simulink model "CurrentSystem2019a"  (R2019a)
settings: Solver=ode23tb  StartTime=0  StopTime=24*365*60*60  RelTol=0.1  EnableMultiTasking=on
PreLoadFcn:
  | power_13NodeTestFeeder_init;
undefined symbols (not defined in the file): ABSOLARCap, ABWindCap, BCSOLARCap, BCWindCap, C_601, C_602, C_603, C_604, C_605, C_606, C_607, ft2km, L_601, L_602, L_603, L_604, L_605, L_606, L_607, MBSOLARCap, MBWindCap, NBSOLARCap, NBWindCap, NLSOLARCap, NLWindCap, NSSOLARCap, NSWindCap, NTSOLARCap, NTWindCap, NUSOLARCap, NUWindCap, ONSOLARCap, ONWindCap, PEISOLARCap, PEIWindCap, QCSOLARCap, QCWindCap, R_601, R_602, R_603, R_604, R_605, R_606, R_607, SKSOLARCap, SKWindCap, T_Disconnect, T_Reconnect, Yearsec, YTSOLARCap, YTWindCap
libraries: powerlib_meascontrol x70, powerlib x67, sps_avr x1, spsDieselMotorModel x1
(part 2 of 3)

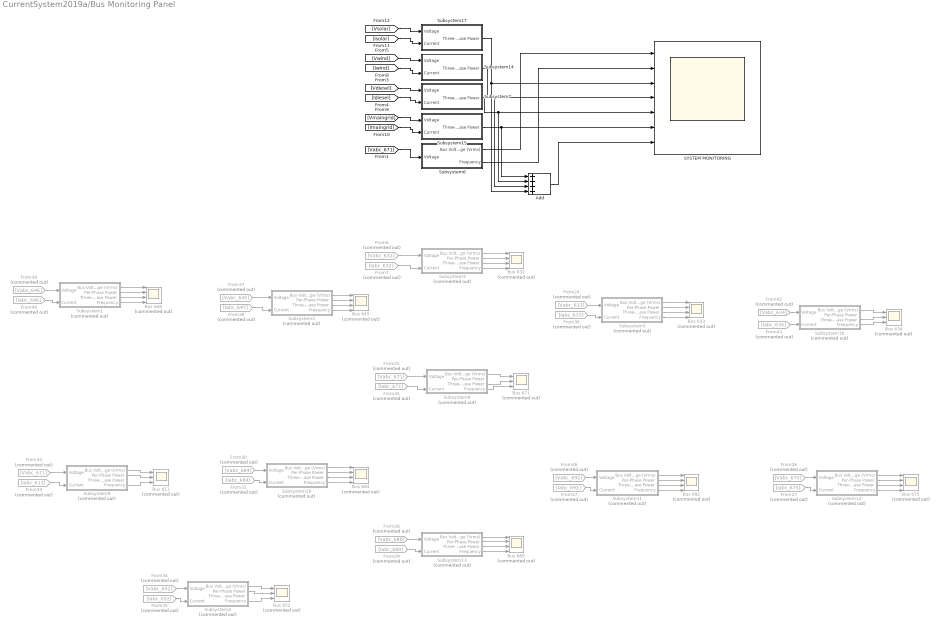
== system CurrentSystem2019a/Bus Monitoring Panel ==
  Add : Sum  Inputs=++++
  Bus {611,634,652,671} (4 alike) : Scope  Commented=on  NumInputPorts=3
  Bus {632..633,645..646,675,680,684,692} (8 alike) : Scope  Commented=on  NumInputPorts=4
  From24 : From  Commented=on  GotoTag=Vabc_633  TagVisibility=global
  From25 : From  Commented=on  GotoTag=Vabc_671  TagVisibility=global
  From26 : From  Commented=on  GotoTag=Vabc_675  TagVisibility=global
  From27 : From  Commented=on  GotoTag=Iabc_675  TagVisibility=global
  From28 : From  Commented=on  GotoTag=Vabc_680  TagVisibility=global
  From29 : From  Commented=on  GotoTag=Iabc_680  TagVisibility=global
  From30 : From  Commented=on  GotoTag=Vabc_684  TagVisibility=global
  From31 : From  Commented=on  GotoTag=Iabc_684  TagVisibility=global
  From32 : From  Commented=on  GotoTag=Vabc_611  TagVisibility=global
  From33 : From  Commented=on  GotoTag=Iabc_611  TagVisibility=global
  From34 : From  Commented=on  GotoTag=Vabc_652  TagVisibility=global
  From35 : From  Commented=on  GotoTag=Iabc_652  TagVisibility=global
  From36 : From  Commented=on  GotoTag=Iabc_633  TagVisibility=global
  From37 : From  Commented=on  GotoTag=Vabc_645  TagVisibility=global
  From38 : From  Commented=on  GotoTag=Iabc_645  TagVisibility=global
  From39 : From  Commented=on  GotoTag=Vabc_646  TagVisibility=global
  From40 : From  Commented=on  GotoTag=Iabc_646  TagVisibility=global
  From41 : From  Commented=on  GotoTag=Iabc_671  TagVisibility=global
  From42 : From  Commented=on  GotoTag=Vabc_634  TagVisibility=global
  From43 : From  Commented=on  GotoTag=Iabc_634  TagVisibility=global
  From46 : From  Commented=on  GotoTag=Vabc_692  TagVisibility=global
  From47 : From  Commented=on  GotoTag=Iabc_692  TagVisibility=global
  From6 : From  Commented=on  GotoTag=Vabc_632  TagVisibility=global
  From7 : From  Commented=on  GotoTag=Iabc_632  TagVisibility=global
  SYSTEM MONITORING : Scope  NumInputPorts=7
  Subsystem1 : Subsystem  Commented=on
  Subsystem10 : Subsystem  Commented=on
  Subsystem11 : Subsystem  Commented=on
  Subsystem12 : Subsystem  Commented=on
  Subsystem13 : Subsystem  Commented=on
  Subsystem14 : Subsystem
  Subsystem15 : Subsystem
  Subsystem16 : Subsystem  Commented=on
  Subsystem17 : Subsystem
  Subsystem2 : Subsystem  Commented=on
  Subsystem3 : Subsystem  Commented=on
  Subsystem4 : Subsystem  Commented=on
  Subsystem5 : Subsystem  Commented=on
  Subsystem6 : Subsystem
  Subsystem7 : Subsystem
  Subsystem8 : Subsystem  Commented=on
  Subsystem9 : Subsystem  Commented=on
  wires:
  From37/1 -> Subsystem2/1(Voltage)
  From43/1 -> Subsystem16/2(Current)
  From42/1 -> Subsystem16/1(Voltage)
  Subsystem5/3(Three-Phase Power) -> Bus 633/3
  Subsystem5/1(Bus Voltage (Vrms)) -> Bus 633/1
  Subsystem5/2(Per-Phase Power) -> Bus 633/2
  Subsystem5/4(Frequency) -> Bus 633/4
  From24/1 -> Subsystem5/1(Voltage)
  From36/1 -> Subsystem5/2(Current)
  Subsystem3/4(Frequency) -> Bus 632/4
  Subsystem3/1(Bus Voltage (Vrms)) -> Bus 632/1
  Subsystem3/2(Per-Phase Power) -> Bus 632/2
  Subsystem3/3(Three-Phase Power) -> Bus 632/3
  From6/1 -> Subsystem3/1(Voltage)
  From7/1 -> Subsystem3/2(Current)
  Subsystem2/4(Frequency) -> Bus 645/4
  Subsystem2/1(Bus Voltage (Vrms)) -> Bus 645/1
  Subsystem2/2(Per-Phase Power) -> Bus 645/2
  Subsystem2/3(Three-Phase Power) -> Bus 645/3
  From38/1 -> Subsystem2/2(Current)
  Subsystem1/4(Frequency) -> Bus 646/4
  Subsystem1/1(Bus Voltage (Vrms)) -> Bus 646/1
  Subsystem1/2(Per-Phase Power) -> Bus 646/2
  Subsystem1/3(Three-Phase Power) -> Bus 646/3
  From39/1 -> Subsystem1/1(Voltage)
  From40/1 -> Subsystem1/2(Current)
  From25/1 -> Subsystem8/1(Voltage)
  From41/1 -> Subsystem8/2(Current)
  From32/1 -> Subsystem9/1(Voltage)
  From33/1 -> Subsystem9/2(Current)
  Subsystem10/4(Frequency) -> Bus 684/4
  Subsystem10/1(Bus Voltage (Vrms)) -> Bus 684/1
  Subsystem10/2(Per-Phase Power) -> Bus 684/2
  Subsystem10/3(Three-Phase Power) -> Bus 684/3
  From30/1 -> Subsystem10/1(Voltage)
  From31/1 -> Subsystem10/2(Current)
  Subsystem11/4(Frequency) -> Bus 692/4
  Subsystem11/1(Bus Voltage (Vrms)) -> Bus 692/1
  Subsystem11/2(Per-Phase Power) -> Bus 692/2
  Subsystem11/3(Three-Phase Power) -> Bus 692/3
  From46/1 -> Subsystem11/1(Voltage)
  From47/1 -> Subsystem11/2(Current)
  Subsystem12/4(Frequency) -> Bus 675/4
  Subsystem12/1(Bus Voltage (Vrms)) -> Bus 675/1
  Subsystem12/2(Per-Phase Power) -> Bus 675/2
  Subsystem12/3(Three-Phase Power) -> Bus 675/3
  From26/1 -> Subsystem12/1(Voltage)
  From27/1 -> Subsystem12/2(Current)
  Subsystem13/4(Frequency) -> Bus 680/4
  Subsystem13/1(Bus Voltage (Vrms)) -> Bus 680/1
  Subsystem13/2(Per-Phase Power) -> Bus 680/2
  Subsystem13/3(Three-Phase Power) -> Bus 680/3
  From28/1 -> Subsystem13/1(Voltage)
  From29/1 -> Subsystem13/2(Current)
  From34/1 -> Subsystem4/1(Voltage)
  From35/1 -> Subsystem4/2(Current)
  Subsystem9/1(Bus Voltage (Vrms)) -> Bus 611/1
  Subsystem9/2(Per-Phase Power) -> Bus 611/2
  Subsystem9/4(Frequency) -> Bus 611/3
  Subsystem4/1(Bus Voltage (Vrms)) -> Bus 652/1
  Subsystem4/2(Per-Phase Power) -> Bus 652/2
  Subsystem4/4(Frequency) -> Bus 652/3
  [Vabc_671] -> Subsystem6/1(Voltage)
  Subsystem16/1(Bus Voltage (Vrms)) -> Bus 634/1
  Subsystem16/3(Three-Phase Power) -> Bus 634/2
  Subsystem16/4(Frequency) -> Bus 634/3
  [Idiesel] -> Subsystem7/2(Current)
  [Vdiesel] -> Subsystem7/1(Voltage)
  [Iwind] -> Subsystem14/2(Current)
  [Vwind] -> Subsystem14/1(Voltage)
  Subsystem8/1(Bus Voltage (Vrms)) -> Bus 671/1
  Subsystem8/3(Three-Phase Power) -> Bus 671/2
  Subsystem8/4(Frequency) -> Bus 671/3
  [Vmaingrid] -> Subsystem15/1(Voltage)
  [Imaingrid] -> Subsystem15/2(Current)
  [Isolar] -> Subsystem17/2(Current)
  [Vsolar] -> Subsystem17/1(Voltage)
  Subsystem6/1(Bus Voltage (Vrms)) -> SYSTEM MONITORING/1
  Subsystem6/2(Frequency) -> SYSTEM MONITORING/2
  Subsystem17/1(Three-Phase Power) -> Add/4, SYSTEM MONITORING/3
  Subsystem14/1(Three-Phase Power) -> Add/3, SYSTEM MONITORING/4
  Subsystem7/1(Three-Phase Power) -> Add/2, SYSTEM MONITORING/5
  Subsystem15/1(Three-Phase Power) -> Add/1, SYSTEM MONITORING/6
  Add/1 -> SYSTEM MONITORING/7

== system CurrentSystem2019a/Diesel Generator1 ==
  wref (pu) : Inport
  Vref (pu) : Inport  Port=2
  AC1A Excitation System : sps_avr/AC1A Excitation System  Tr=20e-3  KaTa=[400 .02]  VAminmax=[-14.5 14.5]  VRminmax=[-5.43 6.03]  KfTf=[0.03 1]  TbTc=[0 0]  KeTe=[1 0.8]  Ve12=[4.18 3.14]  SeVe12=[0.1 0.03]  Kd=0.38  Kc=0.2  v0=[1.0249 1.0264]  TsBlock=0
      link override Model/Saturation Vx=Ve*Se[Ve]/Saturation: BeginIndexSearchUsingPreviousIndexResult=on
      settings: SourceProductName=Simscape Electrical  SourceProductBaseCode=PS
  Diesel Engine Governor : spsDieselMotorModel/Diesel Engine Governor  K=29  Tr=[0.01 0.02 0.2]  Ta=[0.25 0.009 0.0384]  Tlim=[0 1.1]  Td=0.024  Pm0=0.050009
      settings: SourceProductName=Simscape Electrical  SourceProductBaseCode=PS
  Generator Measures : Subsystem
  Ground : Ground
  Selected Measurements : Subsystem
  Synchronous Machine : powerlib/Machines/Synchronous Machine pu Standard  PresetModel=No  MechanicalLoad=Mechanical power Pm  ShowDetailedParameters=on  RotorType=Salient-pole  Units=per unit standard parameters  MeasurementBus=off  NominalParameters=[ Pn Vn Fn]  Reactances1=[ 1.81, 0.3, 0.23, 1.76, 0.65, 0.25, 0.15 ]  Reactances2=[1.305 0.296 0.252 0.474 0.243 0.18]  dAxisTimeConstants=Open-circuit  qAxisTimeConstants=Short-circuit  TimeConstants1="[ 4.4849  0.0681  0.1  ]"  TimeConstants2=[ 8.0, 0.03, 1.0, 0.07 ]  TimeConstants3="[  4.49  0.0681  0.0513  ]"  TimeConstants4=[ 8.0, 0.03, 0.3371, 0.0295 ]  TimeConstants5=[ 1.01, 0.053, 0.1 ]  TimeConstants6=[ 1.3201, 0.023, 1.0, 0.07 ]  TimeConstants7=[0.012 0.003 0.003]  TimeConstants8=[ 1.3201, 0.0231, 0.3371, 0.0295 ]  StatorResistance=0.003  Mechanical=[3.7 0 1 ]  PolePairs=20  InitialConditions=[0 -90.7831 0.0390782 0.045527 0.0753264 -35.3217 -89.6639 115.267 1.02644]  SetSaturation=off  Saturation=[0.6404,0.7127,0.8441,0.9214,0.9956,1.082,1.19,1.316,1.457;0.7,0.7698,0.8872,0.9466,0.9969,1.046,1.1,1.151,1.201]  LoadFlowParameters=[1 0 0 0 0]  TsPowergui=0  TsBlock=-1  IterativeModel=Trapezoidal non iterative  IterativeDiscreteModel=Trapezoidal non iterative  BusType=PQ  Pref=Pn*P0  Qref=0  Qmin=-inf  Qmax=inf  PLF=0  QLF=0
      settings: SourceProductName=Simscape Electrical
  A : PMIOPort  Side=Right
  B : PMIOPort  Port=2  Side=Right
  C : PMIOPort  Port=3  Side=Right
  m : Outport
  wires:
  wref (pu)/1 -> Diesel Engine Governor/1
  Diesel Engine Governor/1 -> Synchronous Machine/1
  AC1A Excitation System/1 -> Synchronous Machine/2
  Vref (pu)/1 -> AC1A Excitation System/1
  Synchronous Machine/1 -> Generator Measures/1(m), Selected Measurements/1(m)
  Ground/1 -> AC1A Excitation System/4
  Generator Measures/3(wm) -> Diesel Engine Governor/2
  Generator Measures/2(Vt) -> AC1A Excitation System/2
  Generator Measures/1(Ifd) -> AC1A Excitation System/3
  Selected Measurements/1(sm) -> m/1
  connections:
  A/RConn1 -- Synchronous Machine/RConn1
  B/RConn1 -- Synchronous Machine/RConn2
  C/RConn1 -- Synchronous Machine/RConn3

== system CurrentSystem2019a/MB SOLAR PROFILE ==
  Add : Sum  Inputs=++++++++++++
  Apr : Step  Time=3*Yearsec  After=136-132  SampleTime=0
  Aug : Step  Time=7*Yearsec  After=122-127  SampleTime=0
  Dec : Step  Time=11*Yearsec  After=64-66  SampleTime=0
  Egen : Gain  Gain=MBSOLARCap
  Feb : Step  Time=1*Yearsec  After=106  SampleTime=0
  Jan : Step  Time=1*Yearsec  Before=79  After=0  SampleTime=0
  Jul : Step  Time=6*Yearsec  After=127-124  SampleTime=0
  Jun : Step  Time=5*Yearsec  After=124-127  SampleTime=0
  Mar : Step  Time=2*Yearsec  After=132-106  SampleTime=0
  May : Step  Time=4*Yearsec  After=127-136  SampleTime=0
  Nov : Step  Time=10*Yearsec  After=66-85  SampleTime=0
  Oct : Step  Time=9*Yearsec  After=85-103  SampleTime=0
  Pgen : Gain  Gain=(1/(30*24))*MBSOLARCap
  Sept : Step  Time=8*Yearsec  After=103-122  SampleTime=0
  Energy : Outport
  Power : Outport  Port=2
  wires:
  Dec/1 -> Add/12
  Sept/1 -> Add/9
  Jun/1 -> Add/6
  Nov/1 -> Add/11
  Aug/1 -> Add/8
  Mar/1 -> Add/3
  May/1 -> Add/5
  Apr/1 -> Add/4
  Jan/1 -> Add/1
  Oct/1 -> Add/10
  Jul/1 -> Add/7
  Feb/1 -> Add/2
  Pgen/1 -> Power/1
  Egen/1 -> Energy/1
  Add/1 -> Egen/1, Pgen/1

== system CurrentSystem2019a/MB WIND PROFILE ==
  Add : Sum  Inputs=++++++++++++
  Apr : Step  Time=3*Yearsec  After=165.6-139.2  SampleTime=0
  Aug : Step  Time=7*Yearsec  After=64.8-72  SampleTime=0
  Dec : Step  Time=11*Yearsec  After=127.2-144  SampleTime=0
  Egen : Gain  Gain=MBWindCap
  Feb : Step  Time=1*Yearsec  After=110.4  SampleTime=0
  Jan : Step  Time=1*Yearsec  Before=127.2  After=0  SampleTime=0
  Jul : Step  Time=6*Yearsec  After=72-104.4  SampleTime=0
  Jun : Step  Time=5*Yearsec  After=104.4-127.2  SampleTime=0
  Mar : Step  Time=2*Yearsec  After=139.2-110.4  SampleTime=0
  May : Step  Time=4*Yearsec  After=127.2-165.5  SampleTime=0
  Nov : Step  Time=10*Yearsec  After=144-180  SampleTime=0
  Oct : Step  Time=9*Yearsec  After=180-110.4  SampleTime=0
  Pgen : Gain  Gain=(1/(30*24))*MBWindCap
  Sept : Step  Time=8*Yearsec  After=110.4-64.8  SampleTime=0
  Energy : Outport
  Power : Outport  Port=2
  wires:
  Dec/1 -> Add/12
  Sept/1 -> Add/9
  Jun/1 -> Add/6
  Nov/1 -> Add/11
  Aug/1 -> Add/8
  Mar/1 -> Add/3
  May/1 -> Add/5
  Apr/1 -> Add/4
  Jan/1 -> Add/1
  Oct/1 -> Add/10
  Jul/1 -> Add/7
  Feb/1 -> Add/2
  Pgen/1 -> Power/1
  Egen/1 -> Energy/1
  Add/1 -> Egen/1, Pgen/1

== system CurrentSystem2019a/NB SOLAR PROFILE ==
  Add : Sum  Inputs=++++++++++++
  Apr : Step  Time=3*Yearsec  After=105-113  SampleTime=0
  Aug : Step  Time=7*Yearsec  After=113-112  SampleTime=0
  Dec : Step  Time=11*Yearsec  After=60-60  SampleTime=0
  Egen : Gain  Gain=NBSOLARCap
  Feb : Step  Time=1*Yearsec  After=96  SampleTime=0
  Jan : Step  Time=1*Yearsec  Before=78  After=0  SampleTime=0
  Jul : Step  Time=6*Yearsec  After=112-111  SampleTime=0
  Jun : Step  Time=5*Yearsec  After=111-109  SampleTime=0
  Mar : Step  Time=2*Yearsec  After=113-96  SampleTime=0
  May : Step  Time=4*Yearsec  After=109-105  SampleTime=0
  Nov : Step  Time=10*Yearsec  After=60-83  SampleTime=0
  Oct : Step  Time=9*Yearsec  After=83-103  SampleTime=0
  Pgen : Gain  Gain=(1/(30*24))*NBSOLARCap
  Sept : Step  Time=8*Yearsec  After=103-113  SampleTime=0
  Energy : Outport
  Power : Outport  Port=2
  wires:
  Dec/1 -> Add/12
  Sept/1 -> Add/9
  Jun/1 -> Add/6
  Nov/1 -> Add/11
  Aug/1 -> Add/8
  Mar/1 -> Add/3
  May/1 -> Add/5
  Apr/1 -> Add/4
  Jan/1 -> Add/1
  Oct/1 -> Add/10
  Jul/1 -> Add/7
  Feb/1 -> Add/2
  Pgen/1 -> Power/1
  Egen/1 -> Energy/1
  Add/1 -> Egen/1, Pgen/1

== system CurrentSystem2019a/NB WIND PROFILE ==
  Add : Sum  Inputs=++++++++++++
  Apr : Step  Time=3*Yearsec  After=64.8-91.2  SampleTime=0
  Aug : Step  Time=7*Yearsec  After=0-9.6  SampleTime=0
  Dec : Step  Time=11*Yearsec  After=24-57.6  SampleTime=0
  Egen : Gain  Gain=NBWindCap
  Feb : Step  Time=1*Yearsec  After=50.4  SampleTime=0
  Jan : Step  Time=1*Yearsec  Before=50.4  After=0  SampleTime=0
  Jul : Step  Time=6*Yearsec  After=9.6-24  SampleTime=0
  Jun : Step  Time=5*Yearsec  After=24-60  SampleTime=0
  Mar : Step  Time=2*Yearsec  After=91.2-50.4  SampleTime=0
  May : Step  Time=4*Yearsec  After=60-64.8  SampleTime=0
  Nov : Step  Time=10*Yearsec  After=57.6-24  SampleTime=0
  Oct : Step  Time=9*Yearsec  After=24-9.6  SampleTime=0
  Pgen : Gain  Gain=(1/(30*24))*NBWindCap
  Sept : Step  Time=8*Yearsec  After=9.6-0  SampleTime=0
  Energy : Outport
  Power : Outport  Port=2
  wires:
  Dec/1 -> Add/12
  Sept/1 -> Add/9
  Jun/1 -> Add/6
  Nov/1 -> Add/11
  Aug/1 -> Add/8
  Mar/1 -> Add/3
  May/1 -> Add/5
  Apr/1 -> Add/4
  Jan/1 -> Add/1
  Oct/1 -> Add/10
  Jul/1 -> Add/7
  Feb/1 -> Add/2
  Pgen/1 -> Power/1
  Egen/1 -> Energy/1
  Add/1 -> Egen/1, Pgen/1

== system CurrentSystem2019a/NL SOLAR PROFILE ==
  Add : Sum  Inputs=++++++++++++
  Apr : Step  Time=3*Yearsec  After=96-95  SampleTime=0
  Aug : Step  Time=7*Yearsec  After=99-103  SampleTime=0
  Dec : Step  Time=11*Yearsec  After=38-44  SampleTime=0
  Egen : Gain  Gain=NLSOLARCap
  Feb : Step  Time=1*Yearsec  After=75  SampleTime=0
  Jan : Step  Time=1*Yearsec  Before=51  After=0  SampleTime=0
  Jul : Step  Time=6*Yearsec  After=103-100  SampleTime=0
  Jun : Step  Time=5*Yearsec  After=100-98  SampleTime=0
  Mar : Step  Time=2*Yearsec  After=95-75  SampleTime=0
  May : Step  Time=4*Yearsec  After=98-96  SampleTime=0
  Nov : Step  Time=10*Yearsec  After=44-63  SampleTime=0
  Oct : Step  Time=9*Yearsec  After=63-85  SampleTime=0
  Pgen : Gain  Gain=(1/(30*24))*NLSOLARCap
  Sept : Step  Time=8*Yearsec  After=85-99  SampleTime=0
  Energy : Outport
  Power : Outport  Port=2
  wires:
  Dec/1 -> Add/12
  Sept/1 -> Add/9
  Jun/1 -> Add/6
  Nov/1 -> Add/11
  Aug/1 -> Add/8
  Mar/1 -> Add/3
  May/1 -> Add/5
  Apr/1 -> Add/4
  Jan/1 -> Add/1
  Oct/1 -> Add/10
  Jul/1 -> Add/7
  Feb/1 -> Add/2
  Pgen/1 -> Power/1
  Egen/1 -> Energy/1
  Add/1 -> Egen/1, Pgen/1

== system CurrentSystem2019a/NL WIND PROFILE ==
  Add : Sum  Inputs=++++++++++++
  Apr : Step  Time=3*Yearsec  After=408-420  SampleTime=0
  Aug : Step  Time=7*Yearsec  After=168-216  SampleTime=0
  Dec : Step  Time=11*Yearsec  After=516-336  SampleTime=0
  Egen : Gain  Gain=NLWindCap
  Feb : Step  Time=1*Yearsec  After=552  SampleTime=0
  Jan : Step  Time=1*Yearsec  Before=420  After=0  SampleTime=0
  Jul : Step  Time=6*Yearsec  After=216-264  SampleTime=0
  Jun : Step  Time=5*Yearsec  After=264-264  SampleTime=0
  Mar : Step  Time=2*Yearsec  After=420-552  SampleTime=0
  May : Step  Time=4*Yearsec  After=264-408  SampleTime=0
  Nov : Step  Time=10*Yearsec  After=336-264  SampleTime=0
  Oct : Step  Time=9*Yearsec  After=264-228  SampleTime=0
  Pgen : Gain  Gain=(1/(30*24))*NLWindCap
  Sept : Step  Time=8*Yearsec  After=228-168  SampleTime=0
  Energy : Outport
  Power : Outport  Port=2
  wires:
  Dec/1 -> Add/12
  Sept/1 -> Add/9
  Jun/1 -> Add/6
  Nov/1 -> Add/11
  Aug/1 -> Add/8
  Mar/1 -> Add/3
  May/1 -> Add/5
  Apr/1 -> Add/4
  Jan/1 -> Add/1
  Oct/1 -> Add/10
  Jul/1 -> Add/7
  Feb/1 -> Add/2
  Pgen/1 -> Power/1
  Egen/1 -> Energy/1
  Add/1 -> Egen/1, Pgen/1

== system CurrentSystem2019a/NS SOLAR PROFILE ==
  Add : Sum  Inputs=++++++++++++
  Apr : Step  Time=3*Yearsec  After=98-105  SampleTime=0
  Aug : Step  Time=7*Yearsec  After=111-111  SampleTime=0
  Dec : Step  Time=11*Yearsec  After=52-56  SampleTime=0
  Egen : Gain  Gain=NSSOLARCap
  Feb : Step  Time=1*Yearsec  After=89  SampleTime=0
  Jan : Step  Time=1*Yearsec  Before=66  After=0  SampleTime=0
  Jul : Step  Time=6*Yearsec  After=111-112  SampleTime=0
  Jun : Step  Time=5*Yearsec  After=112-106  SampleTime=0
  Mar : Step  Time=2*Yearsec  After=105-89  SampleTime=0
  May : Step  Time=4*Yearsec  After=106-98  SampleTime=0
  Nov : Step  Time=10*Yearsec  After=56-82  SampleTime=0
  Oct : Step  Time=9*Yearsec  After=82-102  SampleTime=0
  Pgen : Gain  Gain=(1/(30*24))*NSSOLARCap
  Sept : Step  Time=8*Yearsec  After=102-111  SampleTime=0
  Energy : Outport
  Power : Outport  Port=2
  wires:
  Dec/1 -> Add/12
  Sept/1 -> Add/9
  Jun/1 -> Add/6
  Nov/1 -> Add/11
  Aug/1 -> Add/8
  Mar/1 -> Add/3
  May/1 -> Add/5
  Apr/1 -> Add/4
  Jan/1 -> Add/1
  Oct/1 -> Add/10
  Jul/1 -> Add/7
  Feb/1 -> Add/2
  Pgen/1 -> Power/1
  Egen/1 -> Energy/1
  Add/1 -> Egen/1, Pgen/1

== system CurrentSystem2019a/NS WIND PROFILE ==
  Add : Sum  Inputs=++++++++++++
  Apr : Step  Time=3*Yearsec  After=66-96  SampleTime=0
  Aug : Step  Time=7*Yearsec  After=0-0  SampleTime=0
  Dec : Step  Time=11*Yearsec  After=69.6-72  SampleTime=0
  Egen : Gain  Gain=NSWindCap
  Feb : Step  Time=1*Yearsec  After=72  SampleTime=0
  Jan : Step  Time=1*Yearsec  Before=91.2  After=0  SampleTime=0
  Jul : Step  Time=6*Yearsec  After=0-12  SampleTime=0
  Jun : Step  Time=5*Yearsec  After=12-20.4  SampleTime=0
  Mar : Step  Time=2*Yearsec  After=96-72  SampleTime=0
  May : Step  Time=4*Yearsec  After=20.4-66  SampleTime=0
  Nov : Step  Time=10*Yearsec  After=72-45.6  SampleTime=0
  Oct : Step  Time=9*Yearsec  After=45.6-13.2  SampleTime=0
  Pgen : Gain  Gain=(1/(30*24))*NSWindCap
  Sept : Step  Time=8*Yearsec  After=13.2-0  SampleTime=0
  Energy : Outport
  Power : Outport  Port=2
  wires:
  Dec/1 -> Add/12
  Sept/1 -> Add/9
  Jun/1 -> Add/6
  Nov/1 -> Add/11
  Aug/1 -> Add/8
  Mar/1 -> Add/3
  May/1 -> Add/5
  Apr/1 -> Add/4
  Jan/1 -> Add/1
  Oct/1 -> Add/10
  Jul/1 -> Add/7
  Feb/1 -> Add/2
  Pgen/1 -> Power/1
  Egen/1 -> Energy/1
  Add/1 -> Egen/1, Pgen/1

== system CurrentSystem2019a/NT SOLAR PROFILE ==
  Add : Sum  Inputs=++++++++++++
  Apr : Step  Time=3*Yearsec  After=98-105  SampleTime=0
  Aug : Step  Time=7*Yearsec  After=111-111  SampleTime=0
  Dec : Step  Time=11*Yearsec  After=52-56  SampleTime=0
  Egen : Gain  Gain=NTSOLARCap
  Feb : Step  Time=1*Yearsec  After=89  SampleTime=0
  Jan : Step  Time=1*Yearsec  Before=66  After=0  SampleTime=0
  Jul : Step  Time=6*Yearsec  After=111-112  SampleTime=0
  Jun : Step  Time=5*Yearsec  After=112-106  SampleTime=0
  Mar : Step  Time=2*Yearsec  After=105-89  SampleTime=0
  May : Step  Time=4*Yearsec  After=106-98  SampleTime=0
  Nov : Step  Time=10*Yearsec  After=56-82  SampleTime=0
  Oct : Step  Time=9*Yearsec  After=82-102  SampleTime=0
  Pgen : Gain  Gain=(1/(30*24))*NTSOLARCap
  Scope : Scope
  Sept : Step  Time=8*Yearsec  After=102-111  SampleTime=0
  Energy : Outport
  Power : Outport  Port=2
  wires:
  Dec/1 -> Add/12
  Sept/1 -> Add/9
  Jun/1 -> Add/6
  Nov/1 -> Add/11
  Aug/1 -> Add/8
  Mar/1 -> Add/3
  May/1 -> Add/5
  Apr/1 -> Add/4
  Jan/1 -> Add/1
  Oct/1 -> Add/10
  Jul/1 -> Add/7
  Feb/1 -> Add/2
  Pgen/1 -> Power/1
  Egen/1 -> Energy/1
  Add/1 -> Scope/1, Egen/1, Pgen/1

== system CurrentSystem2019a/NT WIND PROFILE ==
  Add : Sum  Inputs=++++++++++++
  Apr : Step  Time=3*Yearsec  After=67.2-52.8  SampleTime=0
  Aug : Step  Time=7*Yearsec  After=52.8-63.6  SampleTime=0
  Dec : Step  Time=11*Yearsec  After=24-60  SampleTime=0
  Egen : Gain  Gain=NTWindCap
  Feb : Step  Time=1*Yearsec  After=24  SampleTime=0
  Jan : Step  Time=1*Yearsec  Before=36  After=0  SampleTime=0
  Jul : Step  Time=6*Yearsec  After=63.6-78  SampleTime=0
  Jun : Step  Time=5*Yearsec  After=78-96  SampleTime=0
  Mar : Step  Time=2*Yearsec  After=52.8-24  SampleTime=0
  May : Step  Time=4*Yearsec  After=96-67.2  SampleTime=0
  Nov : Step  Time=10*Yearsec  After=60-60  SampleTime=0
  Oct : Step  Time=9*Yearsec  After=60-84  SampleTime=0
  Pgen : Gain  Gain=(1/(30*24))*NTWindCap
  Sept : Step  Time=8*Yearsec  After=84-52.8  SampleTime=0
  Energy : Outport
  Power : Outport  Port=2
  wires:
  Dec/1 -> Add/12
  Sept/1 -> Add/9
  Jun/1 -> Add/6
  Nov/1 -> Add/11
  Aug/1 -> Add/8
  Mar/1 -> Add/3
  May/1 -> Add/5
  Apr/1 -> Add/4
  Jan/1 -> Add/1
  Oct/1 -> Add/10
  Jul/1 -> Add/7
  Feb/1 -> Add/2
  Pgen/1 -> Power/1
  Egen/1 -> Energy/1
  Add/1 -> Egen/1, Pgen/1

== system CurrentSystem2019a/NU SOLAR PROFILE ==
  Add : Sum  Inputs=++++++++++++
  Apr : Step  Time=3*Yearsec  After=175-153  SampleTime=0
  Aug : Step  Time=7*Yearsec  After=92-111  SampleTime=0
  Dec : Step  Time=11*Yearsec  After=15-34  SampleTime=0
  Egen : Gain  Gain=NUSOLARCap
  Feb : Step  Time=1*Yearsec  After=89  SampleTime=0
  Jan : Step  Time=1*Yearsec  Before=31  After=0  SampleTime=0
  Jul : Step  Time=6*Yearsec  After=111-126  SampleTime=0
  Jun : Step  Time=5*Yearsec  After=126-153  SampleTime=0
  Mar : Step  Time=2*Yearsec  After=153-89  SampleTime=0
  May : Step  Time=4*Yearsec  After=153-175  SampleTime=0
  Nov : Step  Time=10*Yearsec  After=34-51  SampleTime=0
  Oct : Step  Time=9*Yearsec  After=51-64  SampleTime=0
  Pgen : Gain  Gain=(1/(30*24))*NUSOLARCap
  Sept : Step  Time=8*Yearsec  After=64-92  SampleTime=0
  Energy : Outport
  Power : Outport  Port=2
  wires:
  Dec/1 -> Add/12
  Sept/1 -> Add/9
  Jun/1 -> Add/6
  Nov/1 -> Add/11
  Aug/1 -> Add/8
  Mar/1 -> Add/3
  May/1 -> Add/5
  Apr/1 -> Add/4
  Jan/1 -> Add/1
  Oct/1 -> Add/10
  Jul/1 -> Add/7
  Feb/1 -> Add/2
  Pgen/1 -> Power/1
  Egen/1 -> Energy/1
  Add/1 -> Egen/1, Pgen/1

== system CurrentSystem2019a/NU WIND PROFILE ==
  Add : Sum  Inputs=++++++++++++
  Apr : Step  Time=3*Yearsec  After=204-168  SampleTime=0
  Aug : Step  Time=7*Yearsec  After=52.8-60  SampleTime=0
  Dec : Step  Time=11*Yearsec  After=105.6-122.4  SampleTime=0
  Egen : Gain  Gain=NUWindCap
  Feb : Step  Time=1*Yearsec  After=100.8  SampleTime=0
  Jan : Step  Time=1*Yearsec  Before=96  After=0  SampleTime=0
  Jul : Step  Time=6*Yearsec  After=60-67.2  SampleTime=0
  Jun : Step  Time=5*Yearsec  After=67.2-108  SampleTime=0
  Mar : Step  Time=2*Yearsec  After=168-100.8  SampleTime=0
  May : Step  Time=4*Yearsec  After=108-204  SampleTime=0
  Nov : Step  Time=10*Yearsec  After=122.4-104.4  SampleTime=0
  Oct : Step  Time=9*Yearsec  After=104.4-100.8  SampleTime=0
  Pgen : Gain  Gain=(1/(30*24))*NUWindCap
  Sept : Step  Time=8*Yearsec  After=100.8-52.8  SampleTime=0
  Energy : Outport
  Power : Outport  Port=2
  wires:
  Dec/1 -> Add/12
  Sept/1 -> Add/9
  Jun/1 -> Add/6
  Nov/1 -> Add/11
  Aug/1 -> Add/8
  Mar/1 -> Add/3
  May/1 -> Add/5
  Apr/1 -> Add/4
  Jan/1 -> Add/1
  Oct/1 -> Add/10
  Jul/1 -> Add/7
  Feb/1 -> Add/2
  Pgen/1 -> Power/1
  Egen/1 -> Energy/1
  Add/1 -> Egen/1, Pgen/1

== system CurrentSystem2019a/ON SOLAR PROFILE ==
  Add : Sum  Inputs=++++++++++++
  Apr : Step  Time=3*Yearsec  After=115-109  SampleTime=0
  Aug : Step  Time=7*Yearsec  After=118-125  SampleTime=0
  Dec : Step  Time=11*Yearsec  After=52-56  SampleTime=0
  Egen : Gain  Gain=ONSOLARCap
  Feb : Step  Time=1*Yearsec  After=92  SampleTime=0
  Jan : Step  Time=1*Yearsec  Before=66  After=0  SampleTime=0
  Jul : Step  Time=6*Yearsec  After=125-124  SampleTime=0
  Jun : Step  Time=5*Yearsec  After=124-119  SampleTime=0
  Mar : Step  Time=2*Yearsec  After=109-92  SampleTime=0
  May : Step  Time=4*Yearsec  After=119-115  SampleTime=0
  Nov : Step  Time=10*Yearsec  After=56-86  SampleTime=0
  Oct : Step  Time=9*Yearsec  After=86-104  SampleTime=0
  Pgen : Gain  Gain=(1/(30*24))*ONSOLARCap
  Sept : Step  Time=8*Yearsec  After=104-118  SampleTime=0
  Energy : Outport
  Power : Outport  Port=2
  wires:
  Dec/1 -> Add/12
  Sept/1 -> Add/9
  Jun/1 -> Add/6
  Nov/1 -> Add/11
  Aug/1 -> Add/8
  Mar/1 -> Add/3
  May/1 -> Add/5
  Apr/1 -> Add/4
  Jan/1 -> Add/1
  Oct/1 -> Add/10
  Jul/1 -> Add/7
  Feb/1 -> Add/2
  Pgen/1 -> Power/1
  Egen/1 -> Energy/1
  Add/1 -> Egen/1, Pgen/1

== system CurrentSystem2019a/ON WIND PROFILE ==
  Add : Sum  Inputs=++++++++++++
  Apr : Step  Time=3*Yearsec  After=110.4-127.2  SampleTime=0
  Aug : Step  Time=7*Yearsec  After=63.6-67.2  SampleTime=0
  Dec : Step  Time=11*Yearsec  After=110.4-105.6  SampleTime=0
  Egen : Gain  Gain=ONWindCap
  Feb : Step  Time=1*Yearsec  After=160.8  SampleTime=0
  Jan : Step  Time=1*Yearsec  Before=144  After=0  SampleTime=0
  Jul : Step  Time=6*Yearsec  After=67.2-91.2  SampleTime=0
  Jun : Step  Time=5*Yearsec  After=91.2-88.8  SampleTime=0
  Mar : Step  Time=2*Yearsec  After=127.2-160.8  SampleTime=0
  May : Step  Time=4*Yearsec  After=88.8-110.4  SampleTime=0
  Nov : Step  Time=10*Yearsec  After=105.6-96  SampleTime=0
  Oct : Step  Time=9*Yearsec  After=96-60  SampleTime=0
  Pgen : Gain  Gain=(1/(30*24))*ONWindCap
  Sept : Step  Time=8*Yearsec  After=60-63.6  SampleTime=0
  Energy : Outport
  Power : Outport  Port=2
  wires:
  Dec/1 -> Add/12
  Sept/1 -> Add/9
  Jun/1 -> Add/6
  Nov/1 -> Add/11
  Aug/1 -> Add/8
  Mar/1 -> Add/3
  May/1 -> Add/5
  Apr/1 -> Add/4
  Jan/1 -> Add/1
  Oct/1 -> Add/10
  Jul/1 -> Add/7
  Feb/1 -> Add/2
  Pgen/1 -> Power/1
  Egen/1 -> Energy/1
  Add/1 -> Egen/1, Pgen/1

== system CurrentSystem2019a/PEI SOLAR PROFILE ==
  Add : Sum  Inputs=++++++++++++
  Apr : Step  Time=3*Yearsec  After=102-110  SampleTime=0
  Aug : Step  Time=7*Yearsec  After=112-114  SampleTime=0
  Dec : Step  Time=11*Yearsec  After=50-54  SampleTime=0
  Egen : Gain  Gain=PEISOLARCap
  Feb : Step  Time=1*Yearsec  After=94  SampleTime=0
  Jan : Step  Time=1*Yearsec  Before=69  After=0  SampleTime=0
  Jul : Step  Time=6*Yearsec  After=114-114  SampleTime=0
  Jun : Step  Time=5*Yearsec  After=114-109  SampleTime=0
  Mar : Step  Time=2*Yearsec  After=110-94  SampleTime=0
  May : Step  Time=4*Yearsec  After=109-102  SampleTime=0
  Nov : Step  Time=10*Yearsec  After=54-77  SampleTime=0
  Oct : Step  Time=9*Yearsec  After=77-100  SampleTime=0
  Pgen : Gain  Gain=(1/(30*24))*PEISOLARCap
  Sept : Step  Time=8*Yearsec  After=100-112  SampleTime=0
  Energy : Outport
  Power : Outport  Port=2
  wires:
  Dec/1 -> Add/12
  Sept/1 -> Add/9
  Jun/1 -> Add/6
  Nov/1 -> Add/11
  Aug/1 -> Add/8
  Mar/1 -> Add/3
  May/1 -> Add/5
  Apr/1 -> Add/4
  Jan/1 -> Add/1
  Oct/1 -> Add/10
  Jul/1 -> Add/7
  Feb/1 -> Add/2
  Pgen/1 -> Power/1
  Egen/1 -> Energy/1
  Add/1 -> Egen/1, Pgen/1

== system CurrentSystem2019a/PEI WIND PROFILE ==
  Add : Sum  Inputs=++++++++++++
  Apr : Step  Time=3*Yearsec  After=120-163.2  SampleTime=0
  Aug : Step  Time=7*Yearsec  After=64.8-64.8  SampleTime=0
  Dec : Step  Time=11*Yearsec  After=120-163.2  SampleTime=0
  Egen : Gain  Gain=PEIWindCap
  Feb : Step  Time=1*Yearsec  After=160.8  SampleTime=0
  Jan : Step  Time=1*Yearsec  Before=144  After=0  SampleTime=0
  Jul : Step  Time=6*Yearsec  After=64.8-100.8  SampleTime=0
  Jun : Step  Time=5*Yearsec  After=100.8-100.8  SampleTime=0
  Mar : Step  Time=2*Yearsec  After=163.2-160.8  SampleTime=0
  May : Step  Time=4*Yearsec  After=100.8-120  SampleTime=0
  Nov : Step  Time=10*Yearsec  After=163.2-98.4  SampleTime=0
  Oct : Step  Time=9*Yearsec  After=98.4-69.6  SampleTime=0
  Pgen : Gain  Gain=(1/(30*24))*PEIWindCap
  Sept : Step  Time=8*Yearsec  After=69.6-64.8  SampleTime=0
  Energy : Outport
  Power : Outport  Port=2
  wires:
  Dec/1 -> Add/12
  Sept/1 -> Add/9
  Jun/1 -> Add/6
  Nov/1 -> Add/11
  Aug/1 -> Add/8
  Mar/1 -> Add/3
  May/1 -> Add/5
  Apr/1 -> Add/4
  Jan/1 -> Add/1
  Oct/1 -> Add/10
  Jul/1 -> Add/7
  Feb/1 -> Add/2
  Pgen/1 -> Power/1
  Egen/1 -> Energy/1
  Add/1 -> Egen/1, Pgen/1

== system CurrentSystem2019a/QC SOLAR PROFILE ==
  Add : Sum  Inputs=++++++++++++
  Apr : Step  Time=3*Yearsec  After=118-124  SampleTime=0
  Aug : Step  Time=7*Yearsec  After=114-117  SampleTime=0
  Dec : Step  Time=11*Yearsec  After=60-59  SampleTime=0
  Egen : Gain  Gain=QCSOLARCap
  Feb : Step  Time=1*Yearsec  After=106  SampleTime=0
  Jan : Step  Time=1*Yearsec  Before=76  After=0  SampleTime=0
  Jul : Step  Time=6*Yearsec  After=117-115  SampleTime=0
  Jun : Step  Time=5*Yearsec  After=115-117  SampleTime=0
  Mar : Step  Time=2*Yearsec  After=124-106  SampleTime=0
  May : Step  Time=4*Yearsec  After=117-118  SampleTime=0
  Nov : Step  Time=10*Yearsec  After=59-80  SampleTime=0
  Oct : Step  Time=9*Yearsec  After=80-98  SampleTime=0
  Pgen : Gain  Gain=(1/(30*24))*QCSOLARCap
  Sept : Step  Time=8*Yearsec  After=98-114  SampleTime=0
  Energy : Outport
  Power : Outport  Port=2
  wires:
  Dec/1 -> Add/12
  Sept/1 -> Add/9
  Jun/1 -> Add/6
  Nov/1 -> Add/11
  Aug/1 -> Add/8
  Mar/1 -> Add/3
  May/1 -> Add/5
  Apr/1 -> Add/4
  Jan/1 -> Add/1
  Oct/1 -> Add/10
  Jul/1 -> Add/7
  Feb/1 -> Add/2
  Pgen/1 -> Power/1
  Egen/1 -> Energy/1
  Add/1 -> Egen/1, Pgen/1

== system CurrentSystem2019a/QC WIND PROFILE ==
  Add : Sum  Inputs=++++++++++++
  Apr : Step  Time=3*Yearsec  After=96-91.2  SampleTime=0
  Aug : Step  Time=7*Yearsec  After=9.6-14.4  SampleTime=0
  Dec : Step  Time=11*Yearsec  After=66-69.6  SampleTime=0
  Egen : Gain  Gain=QCWindCap
  Feb : Step  Time=1*Yearsec  After=103.2  SampleTime=0
  Jan : Step  Time=1*Yearsec  Before=98.4  After=0  SampleTime=0
  Jul : Step  Time=6*Yearsec  After=14.4-50.4  SampleTime=0
  Jun : Step  Time=5*Yearsec  After=50.4-60  SampleTime=0
  Mar : Step  Time=2*Yearsec  After=91.2-103.2  SampleTime=0
  May : Step  Time=4*Yearsec  After=60-96  SampleTime=0
  Nov : Step  Time=10*Yearsec  After=69.6-57.6  SampleTime=0
  Oct : Step  Time=9*Yearsec  After=57.6-11.52  SampleTime=0
  Pgen : Gain  Gain=(1/(30*24))*QCWindCap
  Sept : Step  Time=8*Yearsec  After=11.52-9.6  SampleTime=0
  Energy : Outport
  Power : Outport  Port=2
  wires:
  Dec/1 -> Add/12
  Sept/1 -> Add/9
  Jun/1 -> Add/6
  Nov/1 -> Add/11
  Aug/1 -> Add/8
  Mar/1 -> Add/3
  May/1 -> Add/5
  Apr/1 -> Add/4
  Jan/1 -> Add/1
  Oct/1 -> Add/10
  Jul/1 -> Add/7
  Feb/1 -> Add/2
  Pgen/1 -> Power/1
  Egen/1 -> Energy/1
  Add/1 -> Egen/1, Pgen/1

== system CurrentSystem2019a/SK SOLAR PROFILE ==
  Add : Sum  Inputs=++++++++++++
  Apr : Step  Time=3*Yearsec  After=135-129  SampleTime=0
  Aug : Step  Time=7*Yearsec  After=129-131  SampleTime=0
  Dec : Step  Time=11*Yearsec  After=67-75  SampleTime=0
  Egen : Gain  Gain=SKSOLARCap
  Feb : Step  Time=1*Yearsec  After=111  SampleTime=0
  Jan : Step  Time=1*Yearsec  Before=81  After=0  SampleTime=0
  Jul : Step  Time=6*Yearsec  After=131-128  SampleTime=0
  Jun : Step  Time=5*Yearsec  After=128-128  SampleTime=0
  Mar : Step  Time=2*Yearsec  After=129-111  SampleTime=0
  May : Step  Time=4*Yearsec  After=128-135  SampleTime=0
  Nov : Step  Time=10*Yearsec  After=75-102  SampleTime=0
  Oct : Step  Time=9*Yearsec  After=102-114  SampleTime=0
  Pgen : Gain  Gain=(1/(30*24))*SKSOLARCap
  Sept : Step  Time=8*Yearsec  After=114-129  SampleTime=0
  Energy : Outport
  Power : Outport  Port=2
  wires:
  Dec/1 -> Add/12
  Sept/1 -> Add/9
  Jun/1 -> Add/6
  Nov/1 -> Add/11
  Aug/1 -> Add/8
  Mar/1 -> Add/3
  May/1 -> Add/5
  Apr/1 -> Add/4
  Jan/1 -> Add/1
  Oct/1 -> Add/10
  Jul/1 -> Add/7
  Feb/1 -> Add/2
  Pgen/1 -> Power/1
  Egen/1 -> Energy/1
  Add/1 -> Egen/1, Pgen/1

== system CurrentSystem2019a/SK WIND PROFILE ==
  Add : Sum  Inputs=++++++++++++
  Apr : Step  Time=3*Yearsec  After=204-192  SampleTime=0
  Aug : Step  Time=7*Yearsec  After=88.8-100.8  SampleTime=0
  Dec : Step  Time=11*Yearsec  After=108-127.2  SampleTime=0
  Egen : Gain  Gain=SKWindCap
  Feb : Step  Time=1*Yearsec  After=96  SampleTime=0
  Jan : Step  Time=1*Yearsec  Before=144  After=0  SampleTime=0
  Jul : Step  Time=6*Yearsec  After=100.8-127.2  SampleTime=0
  Jun : Step  Time=5*Yearsec  After=127.2-163.2  SampleTime=0
  Mar : Step  Time=2*Yearsec  After=192-96  SampleTime=0
  May : Step  Time=4*Yearsec  After=163.2-204  SampleTime=0
  Nov : Step  Time=10*Yearsec  After=127.2-160.8  SampleTime=0
  Oct : Step  Time=9*Yearsec  After=160.8-104.4  SampleTime=0
  Pgen : Gain  Gain=(1/(30*24))*SKWindCap
  Sept : Step  Time=8*Yearsec  After=104.4-88.8  SampleTime=0
  Energy : Outport
  Power : Outport  Port=2
  wires:
  Dec/1 -> Add/12
  Sept/1 -> Add/9
  Jun/1 -> Add/6
  Nov/1 -> Add/11
  Aug/1 -> Add/8
  Mar/1 -> Add/3
  May/1 -> Add/5
  Apr/1 -> Add/4
  Jan/1 -> Add/1
  Oct/1 -> Add/10
  Jul/1 -> Add/7
  Feb/1 -> Add/2
  Pgen/1 -> Power/1
  Egen/1 -> Energy/1
  Add/1 -> Egen/1, Pgen/1

== system CurrentSystem2019a/Solar Array ==
  P : Inport
  Bus Selector : BusSelector  OutputSignals=Active power P (W)
  Constant11 : Constant  Value=0
  Mux1 : Mux  Inputs=2
  Simple Solar Inverter : powerlib/Elements/Three-Phase Dynamic Load  NominalVoltage=[Vn Fn]  ActiveReactivePowers=[-250000 -3.38813e-13]  PositiveSequence=[0.999844 -0.0038635]  ExternalControl=on  NpNq=[1.3 2]  TimeConstants="[0  0  0  0]"  MinimumVoltage=0.7  Tfilter=1e-2  LoadFlowParameters=[4,0,0,0,0]
      settings: SourceProductName=Simscape Electrical  SourceProductBaseCode=PS
  Unary Minus : UnaryMinus
  Unary Minus1 : UnaryMinus
  A : PMIOPort  Side=Right
  B : PMIOPort  Port=2  Side=Right
  C : PMIOPort  Port=3  Side=Right
  m : Outport
  wires:
  P/1 -> Unary Minus/1
  Unary Minus/1 -> Mux1/1
  Mux1/1 -> Simple Solar Inverter/1
  Constant11/1 -> Mux1/2
  Simple Solar Inverter/1 -> Bus Selector/1
  Bus Selector/1 -> Unary Minus1/1  "<Active power P (W)>"
  Unary Minus1/1 -> m/1
  connections:
  Simple Solar Inverter/LConn2 -- B/RConn1
  Simple Solar Inverter/LConn3 -- C/RConn1
  Simple Solar Inverter/LConn1 -- A/RConn1

== system CurrentSystem2019a/Wind Turbine ==
  P : Inport
  Bus Selector : BusSelector  OutputSignals=Active power P (W)
  Constant11 : Constant  Value=0
  Mux1 : Mux  Inputs=2
  Simple Solar Inverter : powerlib/Elements/Three-Phase Dynamic Load  NominalVoltage=[Vn Fn]  ActiveReactivePowers=[-250000 -3.38813e-13]  PositiveSequence=[0.999844 -0.0038635]  ExternalControl=on  NpNq=[1.3 2]  TimeConstants="[0  0  0  0]"  MinimumVoltage=0.7  Tfilter=1e-2  LoadFlowParameters=[4,0,0,0,0]
      settings: SourceProductName=Simscape Electrical  SourceProductBaseCode=PS
  Unary Minus : UnaryMinus
  Unary Minus1 : UnaryMinus
  A : PMIOPort  Side=Right
  B : PMIOPort  Port=2  Side=Right
  C : PMIOPort  Port=3  Side=Right
  m : Outport
  wires:
  P/1 -> Unary Minus/1
  Unary Minus/1 -> Mux1/1
  Mux1/1 -> Simple Solar Inverter/1
  Constant11/1 -> Mux1/2
  Simple Solar Inverter/1 -> Bus Selector/1
  Bus Selector/1 -> Unary Minus1/1  "<Active power P (W)>"
  Unary Minus1/1 -> m/1
  connections:
  Simple Solar Inverter/LConn2 -- B/RConn1
  Simple Solar Inverter/LConn3 -- C/RConn1
  Simple Solar Inverter/LConn1 -- A/RConn1

== system CurrentSystem2019a/YT SOLAR PROFILE ==
  Add : Sum  Inputs=++++++++++++
  Apr : Step  Time=3*Yearsec  After=126-108  SampleTime=0
  Aug : Step  Time=7*Yearsec  After=107-110  SampleTime=0
  Dec : Step  Time=11*Yearsec  After=17-30  SampleTime=0
  Egen : Gain  Gain=YTSOLARCap
  Feb : Step  Time=1*Yearsec  After=68  SampleTime=0
  Jan : Step  Time=1*Yearsec  Before=29  After=0  SampleTime=0
  Jul : Step  Time=6*Yearsec  After=110-119  SampleTime=0
  Jun : Step  Time=5*Yearsec  After=119-118  SampleTime=0
  Mar : Step  Time=2*Yearsec  After=108-68  SampleTime=0
  May : Step  Time=4*Yearsec  After=118-126  SampleTime=0
  Nov : Step  Time=10*Yearsec  After=30-52  SampleTime=0
  Oct : Step  Time=9*Yearsec  After=52-82  SampleTime=0
  Pgen : Gain  Gain=(1/(30*24))*YTSOLARCap
  Sept : Step  Time=8*Yearsec  After=82-107  SampleTime=0
  Energy : Outport
  Power : Outport  Port=2
  wires:
  Dec/1 -> Add/12
  Sept/1 -> Add/9
  Jun/1 -> Add/6
  Nov/1 -> Add/11
  Aug/1 -> Add/8
  Mar/1 -> Add/3
  May/1 -> Add/5
  Apr/1 -> Add/4
  Jan/1 -> Add/1
  Oct/1 -> Add/10
  Jul/1 -> Add/7
  Feb/1 -> Add/2
  Pgen/1 -> Power/1
  Egen/1 -> Energy/1
  Add/1 -> Egen/1, Pgen/1

== system CurrentSystem2019a/YT WIND PROFILE ==
  Add : Sum  Inputs=++++++++++++
  Apr : Step  Time=3*Yearsec  After=67.2-60  SampleTime=0
  Aug : Step  Time=7*Yearsec  After=48-9.6  SampleTime=0
  Dec : Step  Time=11*Yearsec  After=96-84  SampleTime=0
  Egen : Gain  Gain=YTWindCap
  Feb : Step  Time=1*Yearsec  After=19.2  SampleTime=0
  Jan : Step  Time=1*Yearsec  Before=72  After=0  SampleTime=0
  Jul : Step  Time=6*Yearsec  After=9.6-19.2  SampleTime=0
  Jun : Step  Time=5*Yearsec  After=19.2-72  SampleTime=0
  Mar : Step  Time=2*Yearsec  After=60-19.2  SampleTime=0
  May : Step  Time=4*Yearsec  After=72-67.2  SampleTime=0
  Nov : Step  Time=10*Yearsec  After=84-54  SampleTime=0
  Oct : Step  Time=9*Yearsec  After=54-24  SampleTime=0
  Pgen : Gain  Gain=(1/(30*24))*YTWindCap
  Sept : Step  Time=8*Yearsec  After=24-48  SampleTime=0
  Energy : Outport
  Power : Outport  Port=2
  wires:
  Dec/1 -> Add/12
  Sept/1 -> Add/9
  Jun/1 -> Add/6
  Nov/1 -> Add/11
  Aug/1 -> Add/8
  Mar/1 -> Add/3
  May/1 -> Add/5
  Apr/1 -> Add/4
  Jan/1 -> Add/1
  Oct/1 -> Add/10
  Jul/1 -> Add/7
  Feb/1 -> Add/2
  Pgen/1 -> Power/1
  Egen/1 -> Energy/1
  Add/1 -> Egen/1, Pgen/1

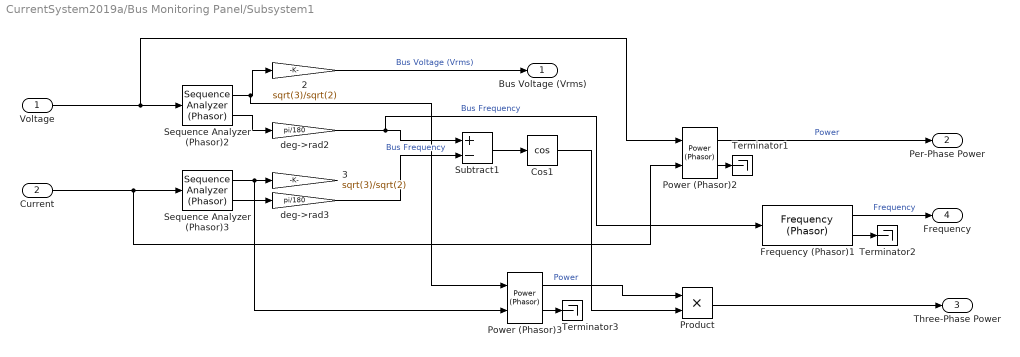
== system CurrentSystem2019a/Bus Monitoring Panel/Subsystem1 ==
  Voltage : Inport
  Current : Inport  Port=2
  " 2" : Gain  Gain=sqrt(3)/sqrt(2)
  " 3" : Gain  Gain=sqrt(3)/sqrt(2)
  Cos1 : Trigonometry  Operator=cos
  Frequency (Phasor)1 : powerlib_meascontrol/Measurements/Frequency (Phasor)  Fn=60  T=0.1
      settings: SourceProductName=Simscape Electrical  SourceProductBaseCode=PS
  Power (Phasor)2 : powerlib_meascontrol/Measurements/Power (Phasor)
      settings: SourceProductName=Simscape Electrical  SourceProductBaseCode=PS
  Power (Phasor)3 : powerlib_meascontrol/Measurements/Power (Phasor)
      settings: SourceProductName=Simscape Electrical  SourceProductBaseCode=PS
  Product : Product
  Sequence Analyzer (Phasor)2 : powerlib_meascontrol/Measurements/Sequence Analyzer (Phasor)  seq=Positive
      settings: SourceProductName=Simscape Electrical  SourceProductBaseCode=PS
  Sequence Analyzer (Phasor)3 : powerlib_meascontrol/Measurements/Sequence Analyzer (Phasor)  seq=Positive
      settings: SourceProductName=Simscape Electrical  SourceProductBaseCode=PS
  Subtract1 : Sum  Inputs=+-
  Terminator1 : Terminator
  Terminator2 : Terminator
  Terminator3 : Terminator
  deg->rad2 : Gain  Gain=pi/180
  deg->rad3 : Gain  Gain=pi/180
  Bus Voltage (Vrms) : Outport  VectorParamsAs1DForOutWhenUnconnected=on
  Per-Phase Power : Outport  Port=2  VectorParamsAs1DForOutWhenUnconnected=on
  Three-Phase Power : Outport  Port=3  VectorParamsAs1DForOutWhenUnconnected=on
  Frequency : Outport  Port=4  VectorParamsAs1DForOutWhenUnconnected=on
  wires:
  Sequence Analyzer (Phasor)2/1 -> Power (Phasor)3/1, " 2"/1
  Sequence Analyzer (Phasor)2/2 -> deg->rad2/1
  Voltage/1 -> Power (Phasor)2/1, Sequence Analyzer (Phasor)2/1
  " 2"/1 -> Bus Voltage (Vrms)/1  "Bus Voltage (Vrms)"
  Sequence Analyzer (Phasor)3/1 -> Power (Phasor)3/2, " 3"/1
  Sequence Analyzer (Phasor)3/2 -> deg->rad3/1
  Current/1 -> Power (Phasor)2/2, Sequence Analyzer (Phasor)3/1
  Subtract1/1 -> Cos1/1
  deg->rad2/1 -> Frequency (Phasor)1/1, Subtract1/1  "Bus Frequency"
  deg->rad3/1 -> Subtract1/2  "Bus Frequency"
  Power (Phasor)2/1 -> Per-Phase Power/1  "Power"
  Power (Phasor)2/2 -> Terminator1/1
  Frequency (Phasor)1/2 -> Terminator2/1
  Frequency (Phasor)1/1 -> Frequency/1  "Frequency"
  Power (Phasor)3/1 -> Product/1  "Power"
  Cos1/1 -> Product/2
  Power (Phasor)3/2 -> Terminator3/1
  Product/1 -> Three-Phase Power/1

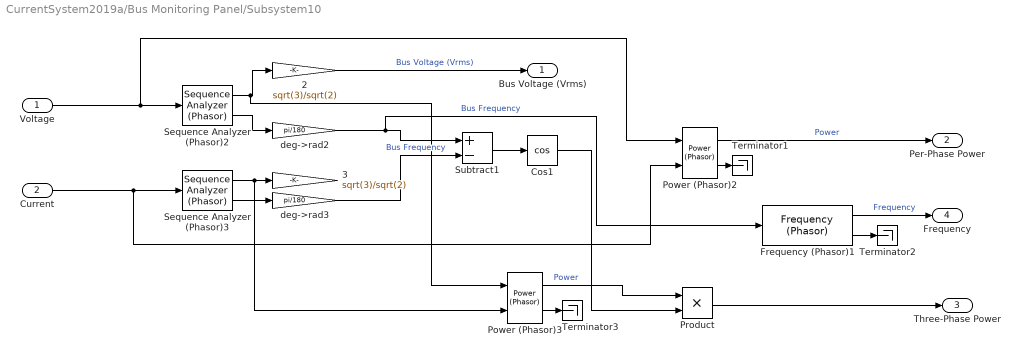
== system CurrentSystem2019a/Bus Monitoring Panel/Subsystem10 ==
  Voltage : Inport
  Current : Inport  Port=2
  " 2" : Gain  Gain=sqrt(3)/sqrt(2)
  " 3" : Gain  Gain=sqrt(3)/sqrt(2)
  Cos1 : Trigonometry  Operator=cos
  Frequency (Phasor)1 : powerlib_meascontrol/Measurements/Frequency (Phasor)  Fn=60  T=0.1
      settings: SourceProductName=Simscape Electrical  SourceProductBaseCode=PS
  Power (Phasor)2 : powerlib_meascontrol/Measurements/Power (Phasor)
      settings: SourceProductName=Simscape Electrical  SourceProductBaseCode=PS
  Power (Phasor)3 : powerlib_meascontrol/Measurements/Power (Phasor)
      settings: SourceProductName=Simscape Electrical  SourceProductBaseCode=PS
  Product : Product
  Sequence Analyzer (Phasor)2 : powerlib_meascontrol/Measurements/Sequence Analyzer (Phasor)  seq=Positive
      settings: SourceProductName=Simscape Electrical  SourceProductBaseCode=PS
  Sequence Analyzer (Phasor)3 : powerlib_meascontrol/Measurements/Sequence Analyzer (Phasor)  seq=Positive
      settings: SourceProductName=Simscape Electrical  SourceProductBaseCode=PS
  Subtract1 : Sum  Inputs=+-
  Terminator1 : Terminator
  Terminator2 : Terminator
  Terminator3 : Terminator
  deg->rad2 : Gain  Gain=pi/180
  deg->rad3 : Gain  Gain=pi/180
  Bus Voltage (Vrms) : Outport  VectorParamsAs1DForOutWhenUnconnected=on
  Per-Phase Power : Outport  Port=2  VectorParamsAs1DForOutWhenUnconnected=on
  Three-Phase Power : Outport  Port=3  VectorParamsAs1DForOutWhenUnconnected=on
  Frequency : Outport  Port=4  VectorParamsAs1DForOutWhenUnconnected=on
  wires:
  Sequence Analyzer (Phasor)2/1 -> Power (Phasor)3/1, " 2"/1
  Sequence Analyzer (Phasor)2/2 -> deg->rad2/1
  Voltage/1 -> Power (Phasor)2/1, Sequence Analyzer (Phasor)2/1
  " 2"/1 -> Bus Voltage (Vrms)/1  "Bus Voltage (Vrms)"
  Sequence Analyzer (Phasor)3/1 -> Power (Phasor)3/2, " 3"/1
  Sequence Analyzer (Phasor)3/2 -> deg->rad3/1
  Current/1 -> Power (Phasor)2/2, Sequence Analyzer (Phasor)3/1
  Subtract1/1 -> Cos1/1
  deg->rad2/1 -> Frequency (Phasor)1/1, Subtract1/1  "Bus Frequency"
  deg->rad3/1 -> Subtract1/2  "Bus Frequency"
  Power (Phasor)2/1 -> Per-Phase Power/1  "Power"
  Power (Phasor)2/2 -> Terminator1/1
  Frequency (Phasor)1/2 -> Terminator2/1
  Frequency (Phasor)1/1 -> Frequency/1  "Frequency"
  Power (Phasor)3/1 -> Product/1  "Power"
  Cos1/1 -> Product/2
  Power (Phasor)3/2 -> Terminator3/1
  Product/1 -> Three-Phase Power/1

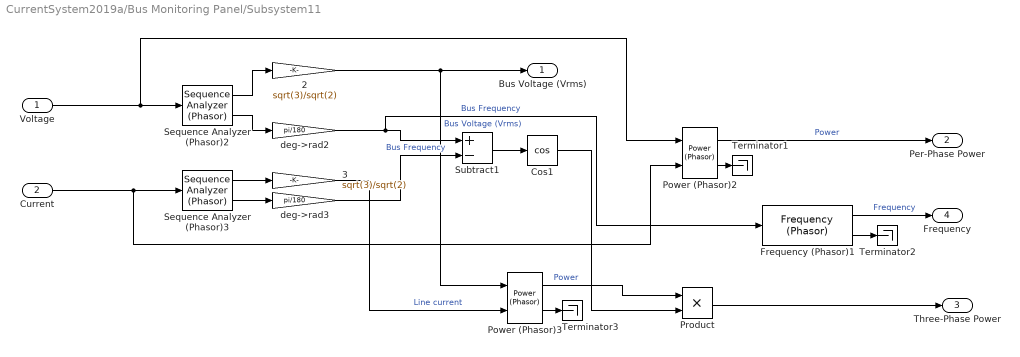
== system CurrentSystem2019a/Bus Monitoring Panel/Subsystem11 ==
  Voltage : Inport
  Current : Inport  Port=2
  " 2" : Gain  Gain=sqrt(3)/sqrt(2)
  " 3" : Gain  Gain=sqrt(3)/sqrt(2)
  Cos1 : Trigonometry  Operator=cos
  Frequency (Phasor)1 : powerlib_meascontrol/Measurements/Frequency (Phasor)  Fn=60  T=0.1
      settings: SourceProductName=Simscape Electrical  SourceProductBaseCode=PS
  Power (Phasor)2 : powerlib_meascontrol/Measurements/Power (Phasor)
      settings: SourceProductName=Simscape Electrical  SourceProductBaseCode=PS
  Power (Phasor)3 : powerlib_meascontrol/Measurements/Power (Phasor)
      settings: SourceProductName=Simscape Electrical  SourceProductBaseCode=PS
  Product : Product
  Sequence Analyzer (Phasor)2 : powerlib_meascontrol/Measurements/Sequence Analyzer (Phasor)  seq=Positive
      settings: SourceProductName=Simscape Electrical  SourceProductBaseCode=PS
  Sequence Analyzer (Phasor)3 : powerlib_meascontrol/Measurements/Sequence Analyzer (Phasor)  seq=Positive
      settings: SourceProductName=Simscape Electrical  SourceProductBaseCode=PS
  Subtract1 : Sum  Inputs=+-
  Terminator1 : Terminator
  Terminator2 : Terminator
  Terminator3 : Terminator
  deg->rad2 : Gain  Gain=pi/180
  deg->rad3 : Gain  Gain=pi/180
  Bus Voltage (Vrms) : Outport  VectorParamsAs1DForOutWhenUnconnected=on
  Per-Phase Power : Outport  Port=2  VectorParamsAs1DForOutWhenUnconnected=on
  Three-Phase Power : Outport  Port=3  VectorParamsAs1DForOutWhenUnconnected=on
  Frequency : Outport  Port=4  VectorParamsAs1DForOutWhenUnconnected=on
  wires:
  Sequence Analyzer (Phasor)2/1 -> " 2"/1
  Sequence Analyzer (Phasor)2/2 -> deg->rad2/1
  Voltage/1 -> Power (Phasor)2/1, Sequence Analyzer (Phasor)2/1
  " 2"/1 -> Power (Phasor)3/1, Bus Voltage (Vrms)/1  "Bus Voltage (Vrms)"
  Sequence Analyzer (Phasor)3/1 -> " 3"/1
  Sequence Analyzer (Phasor)3/2 -> deg->rad3/1
  Current/1 -> Power (Phasor)2/2, Sequence Analyzer (Phasor)3/1
  Subtract1/1 -> Cos1/1
  deg->rad2/1 -> Frequency (Phasor)1/1, Subtract1/1  "Bus Frequency"
  deg->rad3/1 -> Subtract1/2  "Bus Frequency"
  Power (Phasor)2/1 -> Per-Phase Power/1  "Power"
  Power (Phasor)2/2 -> Terminator1/1
  Frequency (Phasor)1/2 -> Terminator2/1
  Frequency (Phasor)1/1 -> Frequency/1  "Frequency"
  " 3"/1 -> Power (Phasor)3/2  "Line current"
  Power (Phasor)3/1 -> Product/1  "Power"
  Cos1/1 -> Product/2
  Power (Phasor)3/2 -> Terminator3/1
  Product/1 -> Three-Phase Power/1

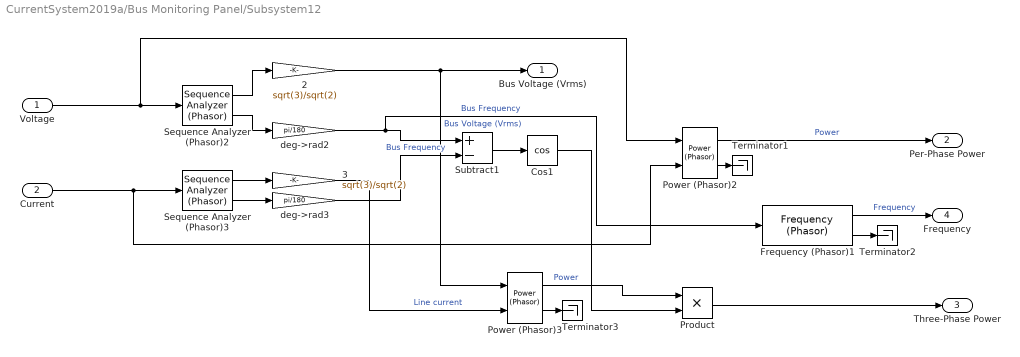
== system CurrentSystem2019a/Bus Monitoring Panel/Subsystem12 ==
  Voltage : Inport
  Current : Inport  Port=2
  " 2" : Gain  Gain=sqrt(3)/sqrt(2)
  " 3" : Gain  Gain=sqrt(3)/sqrt(2)
  Cos1 : Trigonometry  Operator=cos
  Frequency (Phasor)1 : powerlib_meascontrol/Measurements/Frequency (Phasor)  Fn=60  T=0.1
      settings: SourceProductName=Simscape Electrical  SourceProductBaseCode=PS
  Power (Phasor)2 : powerlib_meascontrol/Measurements/Power (Phasor)
      settings: SourceProductName=Simscape Electrical  SourceProductBaseCode=PS
  Power (Phasor)3 : powerlib_meascontrol/Measurements/Power (Phasor)
      settings: SourceProductName=Simscape Electrical  SourceProductBaseCode=PS
  Product : Product
  Sequence Analyzer (Phasor)2 : powerlib_meascontrol/Measurements/Sequence Analyzer (Phasor)  seq=Positive
      settings: SourceProductName=Simscape Electrical  SourceProductBaseCode=PS
  Sequence Analyzer (Phasor)3 : powerlib_meascontrol/Measurements/Sequence Analyzer (Phasor)  seq=Positive
      settings: SourceProductName=Simscape Electrical  SourceProductBaseCode=PS
  Subtract1 : Sum  Inputs=+-
  Terminator1 : Terminator
  Terminator2 : Terminator
  Terminator3 : Terminator
  deg->rad2 : Gain  Gain=pi/180
  deg->rad3 : Gain  Gain=pi/180
  Bus Voltage (Vrms) : Outport  VectorParamsAs1DForOutWhenUnconnected=on
  Per-Phase Power : Outport  Port=2  VectorParamsAs1DForOutWhenUnconnected=on
  Three-Phase Power : Outport  Port=3  VectorParamsAs1DForOutWhenUnconnected=on
  Frequency : Outport  Port=4  VectorParamsAs1DForOutWhenUnconnected=on
  wires:
  Sequence Analyzer (Phasor)2/1 -> " 2"/1
  Sequence Analyzer (Phasor)2/2 -> deg->rad2/1
  Voltage/1 -> Power (Phasor)2/1, Sequence Analyzer (Phasor)2/1
  " 2"/1 -> Power (Phasor)3/1, Bus Voltage (Vrms)/1  "Bus Voltage (Vrms)"
  Sequence Analyzer (Phasor)3/1 -> " 3"/1
  Sequence Analyzer (Phasor)3/2 -> deg->rad3/1
  Current/1 -> Power (Phasor)2/2, Sequence Analyzer (Phasor)3/1
  Subtract1/1 -> Cos1/1
  deg->rad2/1 -> Frequency (Phasor)1/1, Subtract1/1  "Bus Frequency"
  deg->rad3/1 -> Subtract1/2  "Bus Frequency"
  Power (Phasor)2/1 -> Per-Phase Power/1  "Power"
  Power (Phasor)2/2 -> Terminator1/1
  Frequency (Phasor)1/2 -> Terminator2/1
  Frequency (Phasor)1/1 -> Frequency/1  "Frequency"
  " 3"/1 -> Power (Phasor)3/2  "Line current"
  Power (Phasor)3/1 -> Product/1  "Power"
  Cos1/1 -> Product/2
  Power (Phasor)3/2 -> Terminator3/1
  Product/1 -> Three-Phase Power/1
